simulink model "Estimator_soln"  (R2024b)
settings: Solver=VariableStepAuto  StartTime=0.0  StopTime=20.0  MaxStep=.1  RelTol=1e-3
undefined symbols (not defined in the file or in its folder): C, est, K
settings Model: Creator=manand  LastModifiedBy=manand

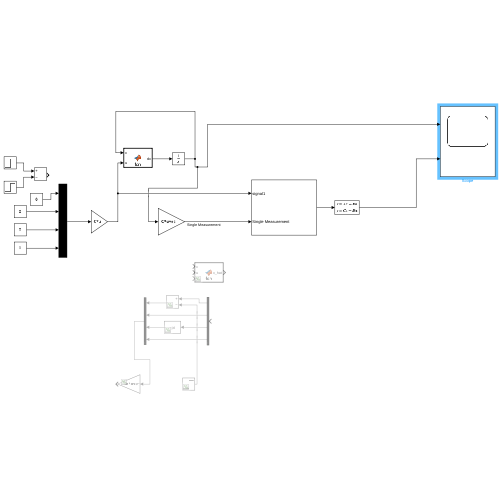
[thumbnail: Simulink's stored preview of the top-level diagram]
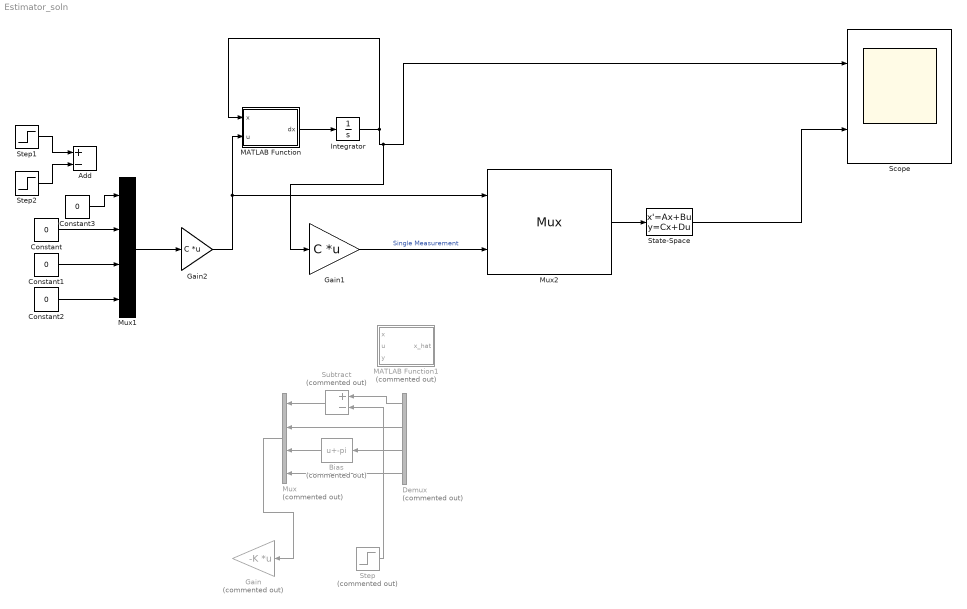
== system Estimator_soln ==
  Add : Sum  Inputs=+-
  Bias : Bias  Commented=on  Bias=-pi  SaturateOnIntegerOverflow=off
  Constant{,1..3} (4 alike) : Constant  Value=0
  Demux : Demux  Commented=on
  Gain : Gain  Commented=on  Gain=-K  Multiplication=Matrix(K*u) (u vector)
  Gain1 : Gain  Gain=C  Multiplication=Matrix(K*u) (u vector)
  Gain2 : Gain  Gain=C  Multiplication=Matrix(K*u)
  Integrator : Integrator  InitialCondition=[0;0;0.1;0]  ZeroCross=off
  MATLAB Function : MATLAB Function  TreatAsAtomicUnit=on
  MATLAB Function1 : MATLAB Function  Commented=on  TreatAsAtomicUnit=on
  Mux : Mux  Commented=on
  Mux1 : Mux
  Mux2 : Mux  Inputs=2
      settings: DisplayOption=signals
  Scope : Scope  NumInputPorts=2
  State-Space : StateSpace  A=est.A  B=est.B  C=est.C  D=est.D  InitialCondition=[0;0;0;0]
  Step : Step  Commented=on  Time=10  SampleTime=0
  Step1 : Step  Time=3  SampleTime=0
  Step2 : Step  Time=4  SampleTime=0
  Subtract : Sum  Commented=on  Inputs=+-
  wires:
  Demux/1 -> Subtract/1
  Demux/3 -> Bias/1
  MATLAB Function/1(dx) -> Integrator/1
  Bias/1 -> Mux/3
  Demux/4 -> Mux/4
  Subtract/1 -> Mux/1
  Mux/1 -> Gain/1
  Demux/2 -> Mux/2
  Step/1 -> Subtract/2
  Integrator/1 -> Scope/1, Gain1/1, MATLAB Function/1(x)
  Constant/1 -> Mux1/2
  Constant1/1 -> Mux1/3
  Constant2/1 -> Mux1/4
  Mux1/1 -> Gain2/1
  Gain2/1 -> MATLAB Function/2(u), Mux2/1
  Step1/1 -> Add/1
  Step2/1 -> Add/2
  Gain1/1 -> Mux2/2  "Single Measurement"
  Mux2/1 -> State-Space/1
  State-Space/1 -> Scope/2
  Constant3/1 -> Mux1/1

== matlab function Estimator_soln/MATLAB Function ==
  data: x input; u input; dx output
function dx = fcn(x,u)
    dx = zeros(4,1);
    m = 1; % mass of pendulum
    M = 5; % mass of cart
    L = 2; % length of pendulum
    g = -9.81; % m/s^2
    d = 1; % Ns/m

  Sx= sin(x(3));
  Cx = cos(x(3));
  D = m*L*L*(M+m*(1-Cx^2));

  dx(1,1) = x(2);
  dx(2,1) = (1/D)*(-m^2*L^2*g*Cx*Sx + m*L^2*(m*L*x(4)^2*Sx-d*x(2)))+m*L^2/D*u;
  dx(3,1) = x(4);
  dx(4,1) = (1/D)*((m+M)*m*g*L*Sx - m*L*Cx*(m*L*x(4)^2*Sx-d*x(2))) - m*L*Cx/D*u;
end

== matlab function Estimator_soln/MATLAB Function1 ==
  data: x input; u input; x_hat output; y input
function x_hat = fcn(x,u,y)
    x_hat = zeros(4,1);
    % m = 1; % mass of pendulum
    % M = 5; % mass of cart
    % L = 2; % length of pendulum
    % g = -9.81; % m/s^2
    % d = 1; % Ns/m

  Sx= sin(x(3));
  Cx = cos(x(3));
  D = m*L*L*(M+m*(1-Cx^2));

  x_hat_dot = (A-Ke'*C)*x_hat+B*u+C*y;
end
